simulink model "Compare_AI_kk"  (R2024b)
settings: Solver=ode1  StartTime=0.0  StopTime=2.5  FixedStep=Ts  RelTol=1e-3
PreLoadFcn:
  | Net_improve_init;L=Lac_MV;Tctrl=Ts;
PostLoadFcn:
  | Net_improve_init;L=Lac_MV;Tctrl=Ts;
InitFcn:
  | Net_improve_init;L=Lac_MV;Tctrl=Ts;
values from neighbouring files (symbols this model uses):
  C1 = 3300e-6    (= 0.0033)    [Net_improve_init.m]
  f_cari = 2e4/4.1    (= 4878.04878049)    [Net_improve_init.m]
  fs = 60    [Net_improve_init.m]
  Lac_MV = 0.005*3    (= 0.015)    [Net_improve_init.m]
  Pref = 0.3e6    (= 300000)    [Net_improve_init.m]
  R1 = 1e-3    (= 0.001)    [Net_improve_init.m]
  Rac_MV = 0.1    [Net_improve_init.m]
  Ts = 20e-6    (= 2e-05)    [Net_improve_init.m]
  Vac_peak_MV = Vref*sqrt(2/3)    [Net_improve_init.m]
  Vdc = 3e3    (= 3000)    [Net_improve_init.m]
undefined symbols (not defined in the file or in its folder): dend, DiscIntNeverNeededParam, numd
libraries: powerlib_extras x15, spsControlledVoltageSourceLib x14, spsCurrentMeasurementLib x8, spsGroundLib x7, spsSeriesRLCBranchLib x7, spsVoltageMeasurementLib x6, spsThreePhaseVIMeasurementLib x5, spsControlledCurrentSourceLib x3, spsIdealSwitchLib x3, spsPower3phInstantaneousLib x3, simulink x3, spsThreePhaseSeriesRLCBranchLib x2
(part 2 of 2)

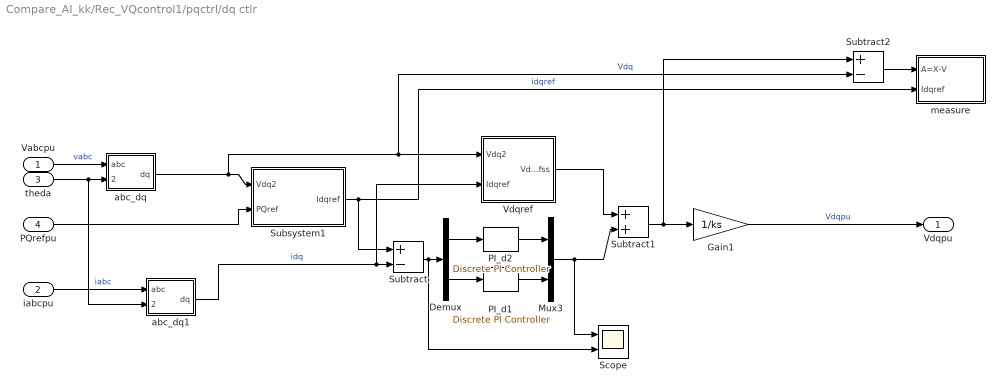
== system Compare_AI_kk/Rec_VQcontrol1/pqctrl/dq ctlr ==
  Vabcpu : Inport
  iabcpu : Inport  Port=2
  theda : Inport  Port=3
  PQrefpu : Inport  Port=4
  Demux : Demux  Outputs=2
  Gain1 : Gain  Gain=1/ks
  Mux3 : Mux  Inputs=2
  PI_d1 : powerlib_extras/Discrete  Control Blocks/Discrete PI Controller  Kp=Kp(1)  Ki=Kp(2)  Par_Limits=[1 -1]*0.15  Init=0  Ts=Ts
  PI_d2 : powerlib_extras/Discrete  Control Blocks/Discrete PI Controller  Kp=Kd(1)  Ki=Kd(2)  Par_Limits=[1 -1]*0.25  Init=0  Ts=Ts
  Scope : Scope  NumInputPorts=2
  Subsystem1 : Subsystem
  Subtract : Sum  Inputs=+-
  Subtract1 : Sum
  Subtract2 : Sum  Inputs=+-
  Vdqref : Subsystem
  abc_dq : Subsystem
  abc_dq1 : Subsystem
  measure : Subsystem
  Vdqpu : Outport  VectorParamsAs1DForOutWhenUnconnected=off
  wires:
  Subtract2/1 -> measure/1(A=X-V)
  Subsystem1/1(Idqref) -> measure/2(Idqref), Subtract/1  "idqref"
  abc_dq/1(dq) -> Subtract2/2, Vdqref/1(Vdq2), Subsystem1/1(Vdq2)  "Vdq"
  abc_dq1/1(dq) -> Vdqref/2(Idqref), Subtract/2  "idq"
  Subtract/1 -> Scope/2, Demux/1
  Demux/1 -> PI_d2/1
  Demux/2 -> PI_d1/1
  Vdqref/1(Vdqrefss) -> Subtract1/1
  PI_d2/1 -> Mux3/1
  PI_d1/1 -> Mux3/2
  Mux3/1 -> Scope/1, Subtract1/2
  Subtract1/1 -> Subtract2/1, Gain1/1
  Vabcpu/1 -> abc_dq/1(abc)  "vabc"
  theda/1 -> abc_dq/2(theta), abc_dq1/2(theta)
  PQrefpu/1 -> Subsystem1/2(PQref)
  iabcpu/1 -> abc_dq1/1(abc)  "iabc"
  Gain1/1 -> Vdqpu/1  "Vdqpu"

== system Compare_AI_kk/Rec_VQcontrol1/pqctrl/dq->abc ==
  note: Va= Vd*sinwt + Vq*cos(wt) + Vo
  note: Vb= Vd*sin(wt-2pi/3) + Vq*cos(wt-2pi/3) + Vo
  note: Vc= Vd*sin(wt+2pi/3) + Vq*cos(wt+2pi/3) + Vo
  dq : Inport
  theda : Inport  Port=2
  Fcn : Fcn  Expr=(u(1)*sin(u(3))+u(2)*cos(u(3)))
  Fcn1 : Fcn  Expr=(u(1)*sin(u(3)-2*pi/3)+u(2)*cos(u(3)-2*pi/3))
  Fcn2 : Fcn  Expr=(u(1)*sin(u(3)+2*pi/3)+u(2)*cos(u(3)+2*pi/3))
  Mux1 : Mux  Inputs=2
  Mux3 : Mux  Inputs=3
  abc : Outport  VectorParamsAs1DForOutWhenUnconnected=off
  wires:
  Fcn2/1 -> Mux3/3
  Fcn1/1 -> Mux3/2
  Fcn/1 -> Mux3/1
  Mux1/1 -> Fcn/1, Fcn2/1, Fcn1/1
  dq/1 -> Mux1/1
  theda/1 -> Mux1/2
  Mux3/1 -> abc/1  "abc"

== system Compare_AI_kk/Rec_VQcontrol1/pqctrl/satuation on amplitute  ==
  Vdq : Inport
  limitVdq : Inport  Port=2
  "Bias important; cancel delay in control cycle, so the PI(error) is zero, other wise PI(errer) is bais, which could over limit" : Bias  Bias=nadv*Ts*2*pi*frq  SaturateOnIntegerOverflow=off
  Complex to Magnitude-Angle : ComplexToMagnitudeAngle
  Complex to Real-Imag : ComplexToRealImag
  Demux1 : Demux  Outputs=2
  Gain : Gain  Gain=-1
  Magnitude-Angle to Complex : MagnitudeAngleToComplex
  Mux4 : Mux  Inputs=2
  Real-Imag to Complex : RealImagToComplex
  Saturation Dynamic : simulink/Discontinuities/Saturation Dynamic  OutMin=[]  OutMax=[]  OutDataTypeStr=Inherit: Same as second input  OutDataType=fixdt(1, 16)  OutScaling=2^-10  DoSatur=off
  Out1 : Outport  VectorParamsAs1DForOutWhenUnconnected=off
  wires:
  "Bias important; cancel delay in control cycle, so the PI(error) is zero, other wise PI(errer) is bais, which could over limit"/1 -> Magnitude-Angle to Complex/2
  Gain/1 -> Saturation Dynamic/3
  limitVdq/1 -> Saturation Dynamic/1, Gain/1
  Complex to Magnitude-Angle/1 -> Saturation Dynamic/2
  Saturation Dynamic/1 -> Magnitude-Angle to Complex/1
  Demux1/1 -> Real-Imag to Complex/1
  Demux1/2 -> Real-Imag to Complex/2
  Real-Imag to Complex/1 -> Complex to Magnitude-Angle/1
  Complex to Magnitude-Angle/2 -> "Bias important; cancel delay in control cycle, so the PI(error) is zero, other wise PI(errer) is bais, which could over limit"/1
  Magnitude-Angle to Complex/1 -> Complex to Real-Imag/1
  Complex to Real-Imag/2 -> Mux4/2
  Complex to Real-Imag/1 -> Mux4/1
  Mux4/1 -> Out1/1
  Vdq/1 -> Demux1/1

== system Compare_AI_kk/Rec_VQcontrol2/Vdc ctrl/Vdc_ctrler1 ==
  Vcap : Inport
  Add2 : Sum  Inputs=+-
  PI_d2 : Subsystem  AncestorBlock=|  DialogController=POWERSYS.PowerSysDialog  mask(Discrete PI Controller){Kp=Kvdc(1), Ki=Kvdc(2), Par_Limits=[1 -1]*1, Init=0, Ts=Ts}
      | powerlib_extras/Discrete 
      | Control Blocks/Discrete
      | PI Controller
      mask prompts: Kp "Proportional gain (Kp):"; Ki "Integral gain (Ki):"; Par_Limits "Output limits: [ Upper   Lower ]"; Init "Output initial value:"; Ts "Sample time:"
      mask help: This block implements a discrete PI controller.
      mask init:
      | UpperLimit=Par_Limits(1);
      | LowerLimit=Par_Limits(2);
      | power_initmask();
      mask Help: This block is part of a subset of blocks in the Extras library that does not have documentation associated with it, other than the block mask description.
      mask Display: disp('PI');
  Saturation : Saturate  UpperLimit=0.1  LowerLimit=-0.1
      settings: AttributesFormatString=%<LowerLimit>~%<UpperLimit>
  Vdcpuref : Constant
  Vdctrl : Scope  NumInputPorts=2
  delP : Outport  OutputWhenDisabled=reset  InitialOutput=[0]  VectorParamsAs1DForOutWhenUnconnected=off
  wires:
  PI_d2/1(Out) -> delP/1, Vdctrl/2  "PIVdc"
  Saturation/1 -> PI_d2/1(Error)
  Vdcpuref/1 -> Add2/2
  Vcap/1 -> Add2/1, Vdctrl/1
  Add2/1 -> Saturation/1  "delVdc"

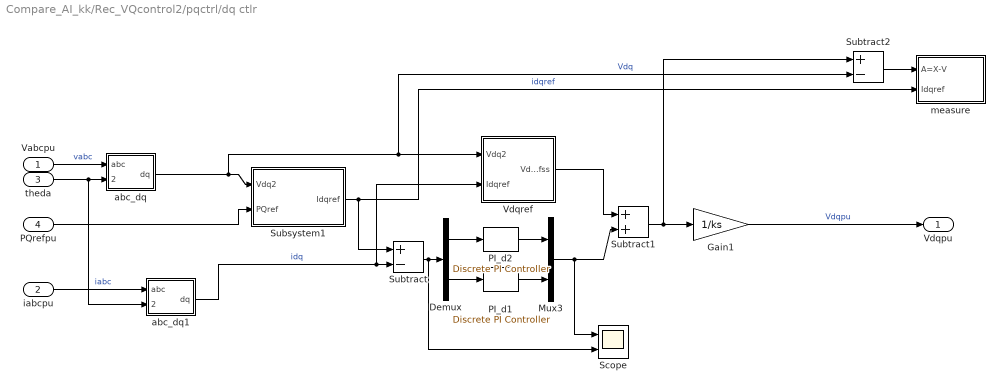
== system Compare_AI_kk/Rec_VQcontrol2/pqctrl/dq ctlr ==
  Vabcpu : Inport
  iabcpu : Inport  Port=2
  theda : Inport  Port=3
  PQrefpu : Inport  Port=4
  Demux : Demux  Outputs=2
  Gain1 : Gain  Gain=1/ks
  Mux3 : Mux  Inputs=2
  PI_d1 : powerlib_extras/Discrete  Control Blocks/Discrete PI Controller  Kp=Kp(1)  Ki=Kp(2)  Par_Limits=[1 -1]*0.15  Init=0  Ts=Ts
  PI_d2 : powerlib_extras/Discrete  Control Blocks/Discrete PI Controller  Kp=Kd(1)  Ki=Kd(2)  Par_Limits=[1 -1]*0.25  Init=0  Ts=Ts
  Scope : Scope  NumInputPorts=2
  Subsystem1 : Subsystem
  Subtract : Sum  Inputs=+-
  Subtract1 : Sum
  Subtract2 : Sum  Inputs=+-
  Vdqref : Subsystem
  abc_dq : Subsystem
  abc_dq1 : Subsystem
  measure : Subsystem
  Vdqpu : Outport  VectorParamsAs1DForOutWhenUnconnected=off
  wires:
  Subtract2/1 -> measure/1(A=X-V)
  Subsystem1/1(Idqref) -> measure/2(Idqref), Subtract/1  "idqref"
  abc_dq/1(dq) -> Subtract2/2, Vdqref/1(Vdq2), Subsystem1/1(Vdq2)  "Vdq"
  abc_dq1/1(dq) -> Vdqref/2(Idqref), Subtract/2  "idq"
  Subtract/1 -> Scope/2, Demux/1
  Demux/1 -> PI_d2/1
  Demux/2 -> PI_d1/1
  Vdqref/1(Vdqrefss) -> Subtract1/1
  PI_d2/1 -> Mux3/1
  PI_d1/1 -> Mux3/2
  Mux3/1 -> Scope/1, Subtract1/2
  Subtract1/1 -> Subtract2/1, Gain1/1
  Vabcpu/1 -> abc_dq/1(abc)  "vabc"
  theda/1 -> abc_dq/2(theta), abc_dq1/2(theta)
  PQrefpu/1 -> Subsystem1/2(PQref)
  iabcpu/1 -> abc_dq1/1(abc)  "iabc"
  Gain1/1 -> Vdqpu/1  "Vdqpu"

== system Compare_AI_kk/Rec_VQcontrol2/pqctrl/dq->abc ==
  note: Va= Vd*sinwt + Vq*cos(wt) + Vo
  note: Vb= Vd*sin(wt-2pi/3) + Vq*cos(wt-2pi/3) + Vo
  note: Vc= Vd*sin(wt+2pi/3) + Vq*cos(wt+2pi/3) + Vo
  dq : Inport
  theda : Inport  Port=2
  Fcn : Fcn  Expr=(u(1)*sin(u(3))+u(2)*cos(u(3)))
  Fcn1 : Fcn  Expr=(u(1)*sin(u(3)-2*pi/3)+u(2)*cos(u(3)-2*pi/3))
  Fcn2 : Fcn  Expr=(u(1)*sin(u(3)+2*pi/3)+u(2)*cos(u(3)+2*pi/3))
  Mux1 : Mux  Inputs=2
  Mux3 : Mux  Inputs=3
  abc : Outport  VectorParamsAs1DForOutWhenUnconnected=off
  wires:
  Fcn2/1 -> Mux3/3
  Fcn1/1 -> Mux3/2
  Fcn/1 -> Mux3/1
  Mux1/1 -> Fcn/1, Fcn2/1, Fcn1/1
  dq/1 -> Mux1/1
  theda/1 -> Mux1/2
  Mux3/1 -> abc/1  "abc"

== system Compare_AI_kk/Rec_VQcontrol2/pqctrl/satuation on amplitute  ==
  Vdq : Inport
  limitVdq : Inport  Port=2
  "Bias important; cancel delay in control cycle, so the PI(error) is zero, other wise PI(errer) is bais, which could over limit" : Bias  Bias=nadv*Ts*2*pi*frq  SaturateOnIntegerOverflow=off
  Complex to Magnitude-Angle : ComplexToMagnitudeAngle
  Complex to Real-Imag : ComplexToRealImag
  Demux1 : Demux  Outputs=2
  Gain : Gain  Gain=-1
  Magnitude-Angle to Complex : MagnitudeAngleToComplex
  Mux4 : Mux  Inputs=2
  Real-Imag to Complex : RealImagToComplex
  Saturation Dynamic : simulink/Discontinuities/Saturation Dynamic  OutMin=[]  OutMax=[]  OutDataTypeStr=Inherit: Same as second input  OutDataType=fixdt(1, 16)  OutScaling=2^-10  DoSatur=off
  Out1 : Outport  VectorParamsAs1DForOutWhenUnconnected=off
  wires:
  "Bias important; cancel delay in control cycle, so the PI(error) is zero, other wise PI(errer) is bais, which could over limit"/1 -> Magnitude-Angle to Complex/2
  Gain/1 -> Saturation Dynamic/3
  limitVdq/1 -> Saturation Dynamic/1, Gain/1
  Complex to Magnitude-Angle/1 -> Saturation Dynamic/2
  Saturation Dynamic/1 -> Magnitude-Angle to Complex/1
  Demux1/1 -> Real-Imag to Complex/1
  Demux1/2 -> Real-Imag to Complex/2
  Real-Imag to Complex/1 -> Complex to Magnitude-Angle/1
  Complex to Magnitude-Angle/2 -> "Bias important; cancel delay in control cycle, so the PI(error) is zero, other wise PI(errer) is bais, which could over limit"/1
  Magnitude-Angle to Complex/1 -> Complex to Real-Imag/1
  Complex to Real-Imag/2 -> Mux4/2
  Complex to Real-Imag/1 -> Mux4/1
  Mux4/1 -> Out1/1
  Vdq/1 -> Demux1/1

== system Compare_AI_kk/Rec_VQcontrol3/Vdc ctrl/Vdc_ctrler1 ==
  Vcap : Inport
  Add2 : Sum  Inputs=+-
  PI_d2 : Subsystem  AncestorBlock=|  DialogController=POWERSYS.PowerSysDialog  mask(Discrete PI Controller){Kp=Kvdc(1), Ki=Kvdc(2), Par_Limits=[1 -1]*1, Init=0, Ts=Ts}
      | powerlib_extras/Discrete 
      | Control Blocks/Discrete
      | PI Controller
      mask prompts: Kp "Proportional gain (Kp):"; Ki "Integral gain (Ki):"; Par_Limits "Output limits: [ Upper   Lower ]"; Init "Output initial value:"; Ts "Sample time:"
      mask help: This block implements a discrete PI controller.
      mask init:
      | UpperLimit=Par_Limits(1);
      | LowerLimit=Par_Limits(2);
      | power_initmask();
      mask Help: This block is part of a subset of blocks in the Extras library that does not have documentation associated with it, other than the block mask description.
      mask Display: disp('PI');
  Saturation : Saturate  UpperLimit=0.1  LowerLimit=-0.1
      settings: AttributesFormatString=%<LowerLimit>~%<UpperLimit>
  Vdcpuref : Constant
  Vdctrl : Scope  NumInputPorts=2
  delP : Outport  OutputWhenDisabled=reset  InitialOutput=[0]  VectorParamsAs1DForOutWhenUnconnected=off
  wires:
  PI_d2/1(Out) -> delP/1, Vdctrl/2  "PIVdc"
  Saturation/1 -> PI_d2/1(Error)
  Vdcpuref/1 -> Add2/2
  Vcap/1 -> Add2/1, Vdctrl/1
  Add2/1 -> Saturation/1  "delVdc"

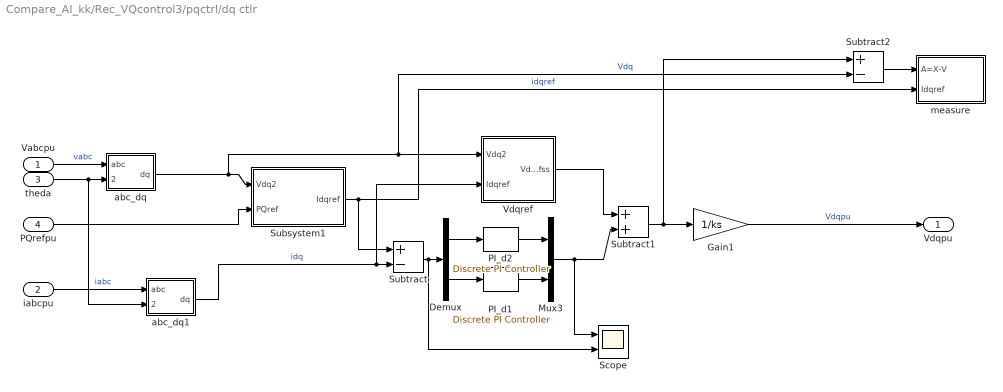
== system Compare_AI_kk/Rec_VQcontrol3/pqctrl/dq ctlr ==
  Vabcpu : Inport
  iabcpu : Inport  Port=2
  theda : Inport  Port=3
  PQrefpu : Inport  Port=4
  Demux : Demux  Outputs=2
  Gain1 : Gain  Gain=1/ks
  Mux3 : Mux  Inputs=2
  PI_d1 : powerlib_extras/Discrete  Control Blocks/Discrete PI Controller  Kp=Kp(1)  Ki=Kp(2)  Par_Limits=[1 -1]*0.15  Init=0  Ts=Ts
  PI_d2 : powerlib_extras/Discrete  Control Blocks/Discrete PI Controller  Kp=Kd(1)  Ki=Kd(2)  Par_Limits=[1 -1]*0.25  Init=0  Ts=Ts
  Scope : Scope  NumInputPorts=2
  Subsystem1 : Subsystem
  Subtract : Sum  Inputs=+-
  Subtract1 : Sum
  Subtract2 : Sum  Inputs=+-
  Vdqref : Subsystem
  abc_dq : Subsystem
  abc_dq1 : Subsystem
  measure : Subsystem
  Vdqpu : Outport  VectorParamsAs1DForOutWhenUnconnected=off
  wires:
  Subtract2/1 -> measure/1(A=X-V)
  Subsystem1/1(Idqref) -> measure/2(Idqref), Subtract/1  "idqref"
  abc_dq/1(dq) -> Subtract2/2, Vdqref/1(Vdq2), Subsystem1/1(Vdq2)  "Vdq"
  abc_dq1/1(dq) -> Vdqref/2(Idqref), Subtract/2  "idq"
  Subtract/1 -> Scope/2, Demux/1
  Demux/1 -> PI_d2/1
  Demux/2 -> PI_d1/1
  Vdqref/1(Vdqrefss) -> Subtract1/1
  PI_d2/1 -> Mux3/1
  PI_d1/1 -> Mux3/2
  Mux3/1 -> Scope/1, Subtract1/2
  Subtract1/1 -> Subtract2/1, Gain1/1
  Vabcpu/1 -> abc_dq/1(abc)  "vabc"
  theda/1 -> abc_dq/2(theta), abc_dq1/2(theta)
  PQrefpu/1 -> Subsystem1/2(PQref)
  iabcpu/1 -> abc_dq1/1(abc)  "iabc"
  Gain1/1 -> Vdqpu/1  "Vdqpu"

== system Compare_AI_kk/Rec_VQcontrol3/pqctrl/dq->abc ==
  note: Va= Vd*sinwt + Vq*cos(wt) + Vo
  note: Vb= Vd*sin(wt-2pi/3) + Vq*cos(wt-2pi/3) + Vo
  note: Vc= Vd*sin(wt+2pi/3) + Vq*cos(wt+2pi/3) + Vo
  dq : Inport
  theda : Inport  Port=2
  Fcn : Fcn  Expr=(u(1)*sin(u(3))+u(2)*cos(u(3)))
  Fcn1 : Fcn  Expr=(u(1)*sin(u(3)-2*pi/3)+u(2)*cos(u(3)-2*pi/3))
  Fcn2 : Fcn  Expr=(u(1)*sin(u(3)+2*pi/3)+u(2)*cos(u(3)+2*pi/3))
  Mux1 : Mux  Inputs=2
  Mux3 : Mux  Inputs=3
  abc : Outport  VectorParamsAs1DForOutWhenUnconnected=off
  wires:
  Fcn2/1 -> Mux3/3
  Fcn1/1 -> Mux3/2
  Fcn/1 -> Mux3/1
  Mux1/1 -> Fcn/1, Fcn2/1, Fcn1/1
  dq/1 -> Mux1/1
  theda/1 -> Mux1/2
  Mux3/1 -> abc/1  "abc"

== system Compare_AI_kk/Rec_VQcontrol3/pqctrl/satuation on amplitute  ==
  Vdq : Inport
  limitVdq : Inport  Port=2
  "Bias important; cancel delay in control cycle, so the PI(error) is zero, other wise PI(errer) is bais, which could over limit" : Bias  Bias=nadv*Ts*2*pi*frq  SaturateOnIntegerOverflow=off
  Complex to Magnitude-Angle : ComplexToMagnitudeAngle
  Complex to Real-Imag : ComplexToRealImag
  Demux1 : Demux  Outputs=2
  Gain : Gain  Gain=-1
  Magnitude-Angle to Complex : MagnitudeAngleToComplex
  Mux4 : Mux  Inputs=2
  Real-Imag to Complex : RealImagToComplex
  Saturation Dynamic : simulink/Discontinuities/Saturation Dynamic  OutMin=[]  OutMax=[]  OutDataTypeStr=Inherit: Same as second input  OutDataType=fixdt(1, 16)  OutScaling=2^-10  DoSatur=off
  Out1 : Outport  VectorParamsAs1DForOutWhenUnconnected=off
  wires:
  "Bias important; cancel delay in control cycle, so the PI(error) is zero, other wise PI(errer) is bais, which could over limit"/1 -> Magnitude-Angle to Complex/2
  Gain/1 -> Saturation Dynamic/3
  limitVdq/1 -> Saturation Dynamic/1, Gain/1
  Complex to Magnitude-Angle/1 -> Saturation Dynamic/2
  Saturation Dynamic/1 -> Magnitude-Angle to Complex/1
  Demux1/1 -> Real-Imag to Complex/1
  Demux1/2 -> Real-Imag to Complex/2
  Real-Imag to Complex/1 -> Complex to Magnitude-Angle/1
  Complex to Magnitude-Angle/2 -> "Bias important; cancel delay in control cycle, so the PI(error) is zero, other wise PI(errer) is bais, which could over limit"/1
  Magnitude-Angle to Complex/1 -> Complex to Real-Imag/1
  Complex to Real-Imag/2 -> Mux4/2
  Complex to Real-Imag/1 -> Mux4/1
  Mux4/1 -> Out1/1
  Vdq/1 -> Demux1/1

== system Compare_AI_kk/Rec_VQcontrol1/Vdc ctrl/Vdc_ctrler1/PI_d2 ==
  note: Discrete PID Controller
  note: Pierre Giroux, Gilbert Sybille
      | Power System Simulation Laboratory
      | IREQ, Hydro-Quebc
  Error : Inport  SampleTime=Ts
  Discrete-Time Integrator : DiscreteIntegrator  InitialCondition=Init  SampleTime=Ts  LimitOutput=on  UpperSaturationLimit=UpperLimit  LowerSaturationLimit=LowerLimit  ICPrevOutput=DiscIntNeverNeededParam  ICPrevScaledInput=DiscIntNeverNeededParam
  Kp4 : Gain  Gain=Kp  SaturateOnIntegerOverflow=on  SampleTime=Ts  OutDataTypeStr=Inherit: Same as input  ParamDataTypeStr=Inherit: Same as input
  Kp5 : Gain  Gain=Ki  SaturateOnIntegerOverflow=on  SampleTime=Ts  OutDataTypeStr=Inherit: Same as input  ParamDataTypeStr=Inherit: Same as input
  Saturation2 : Saturate  UpperLimit=UpperLimit  LowerLimit=LowerLimit  SampleTime=Ts
  Sum6 : Sum  InputSameDT=on  SaturateOnIntegerOverflow=on  SampleTime=Ts  OutDataTypeStr=Inherit: Same as first input
  Zero-Order Hold : ZeroOrderHold  SampleTime=Ts
  Out : Outport  SampleTime=Ts  InitialOutput=0  VectorParamsAs1DForOutWhenUnconnected=off
  wires:
  Zero-Order Hold/1 -> Sum6/1  "prop"
  Saturation2/1 -> Out/1
  Discrete-Time Integrator/1 -> Sum6/2  "int"
  Kp4/1 -> Zero-Order Hold/1
  Kp5/1 -> Discrete-Time Integrator/1
  Sum6/1 -> Saturation2/1
  Error/1 -> Kp5/1, Kp4/1

== system Compare_AI_kk/Rec_VQcontrol1/pqctrl/dq ctlr/Subsystem1 ==
  Vdq2 : Inport
  PQref : Inport  Port=2
  Fcn7 : Fcn  Expr=(u[1] *u[4]+u[2]*u[5])/u[3]
  Fcn8 : Fcn  Expr=(u[2] *u[4]-u[1]*u[5])/u[3]
  Fcn9 : Fcn  Expr=(u[1] ^2+u[2]^2)
  Mux3 : Mux  Inputs=[2 1 2]
  Mux4 : Mux  Inputs=2
  Saturation : Saturate  UpperLimit=inf  LowerLimit=0.01
  Saturation1 : Saturate  UpperLimit=1.5  LowerLimit=-1.5
  Idqref : Outport  VectorParamsAs1DForOutWhenUnconnected=off
  wires:
  Saturation1/1 -> Idqref/1
  Vdq2/1 -> Fcn9/1, Mux3/1
  Mux3/1 -> Fcn8/1, Fcn7/1
  Fcn9/1 -> Saturation/1
  Fcn7/1 -> Mux4/1
  Fcn8/1 -> Mux4/2
  Mux4/1 -> Saturation1/1  "Idqref"
  PQref/1 -> Mux3/3
  Saturation/1 -> Mux3/2

== system Compare_AI_kk/Rec_VQcontrol1/pqctrl/dq ctlr/Vdqref ==
  Vdq2 : Inport
  Idqref : Inport  Port=2
  Display : Display
      settings: Decimation=50
  Fcn7 : Fcn  Expr=(u[2] +u[4]*u[5]+u[3]*u[6])
  Fcn8 : Fcn  Expr=(u[1] +u[3]*u[5]-u[4]*u[6])
  Lxpu : Constant  Value=Lxpu
  Mux3 : Mux
  Mux4 : Mux  Inputs=2
  Rxpu : Constant  Value=Rxpu
  Vdqrefss : Outport  VectorParamsAs1DForOutWhenUnconnected=off
  wires:
  Lxpu/1 -> Mux3/4
  Rxpu/1 -> Mux3/3
  Mux3/1 -> Display/1, Fcn8/1, Fcn7/1
  Fcn8/1 -> Mux4/1  "Vdref"
  Fcn7/1 -> Mux4/2  "Vqref"
  Vdq2/1 -> Mux3/1
  Idqref/1 -> Mux3/2
  Mux4/1 -> Vdqrefss/1

== system Compare_AI_kk/Rec_VQcontrol1/pqctrl/dq ctlr/abc_dq ==
  abc : Inport
  theta : Inport  Port=2
  Mux2 : Mux  Inputs=2
  Selector3 : Selector  InputPortWidth=3  IndexOptions=Index vector (dialog)  Indices=[1 2]  OutputSizes=1
  Trigonometric Function2 : Trigonometry
  Trigonometric Function3 : Trigonometry  Operator=cos
  abc/dq1 : powerlib_extras/Measurements/abc_to_dq0 Transformation
  dq : Outport  VectorParamsAs1DForOutWhenUnconnected=off
  wires:
  abc/1 -> abc/dq1/1
  Selector3/1 -> dq/1
  abc/dq1/1 -> Selector3/1
  Mux2/1 -> abc/dq1/2
  theta/1 -> Trigonometric Function3/1, Trigonometric Function2/1
  Trigonometric Function2/1 -> Mux2/1
  Trigonometric Function3/1 -> Mux2/2

== system Compare_AI_kk/Rec_VQcontrol1/pqctrl/dq ctlr/abc_dq1 ==
  abc : Inport
  theta : Inport  Port=2
  Mux2 : Mux  Inputs=2
  Selector3 : Selector  InputPortWidth=3  IndexOptions=Index vector (dialog)  Indices=[1 2]  OutputSizes=1
  Trigonometric Function2 : Trigonometry
  Trigonometric Function3 : Trigonometry  Operator=cos
  abc/dq1 : powerlib_extras/Measurements/abc_to_dq0 Transformation
  dq : Outport  VectorParamsAs1DForOutWhenUnconnected=off
  wires:
  Trigonometric Function3/1 -> Mux2/2
  Trigonometric Function2/1 -> Mux2/1
  theta/1 -> Trigonometric Function2/1, Trigonometric Function3/1
  Mux2/1 -> abc/dq1/2
  abc/dq1/1 -> Selector3/1
  Selector3/1 -> dq/1
  abc/1 -> abc/dq1/1

== system Compare_AI_kk/Rec_VQcontrol1/pqctrl/dq ctlr/measure ==
  note: this is to validate Rxpu and Lxpu which make PI(error) almost zero,
      | i.e. the delay is properly set
      |
      | or to calculate Rxpu and Lxpu which make PI(error) zero
      | when input are in steady state
      |
      | when change the P,Q ref,
      | the results should be same if delay is properly cancelled
  A=X-V : Inport
  Idqref : Inport  Port=2
  Display1 : Display
      settings: Decimation=200
  Fcn7 : Fcn  Expr=(u[2] *u[3]-u[1]*u[4])/(u[3]^2+u[4]^2)
  Fcn8 : Fcn  Expr=(u[1] *u[3]+u[2]*u[4])/(u[3]^2+u[4]^2)
  Mux3 : Mux  Inputs=2
  Mux4 : Mux  Inputs=2
  wires:
  Mux3/1 -> Fcn8/1, Fcn7/1
  Fcn8/1 -> Mux4/1  "Rxpu"
  Fcn7/1 -> Mux4/2  "Lxpu"
  A=X-V/1 -> Mux3/1
  Idqref/1 -> Mux3/2
  Mux4/1 -> Display1/1

== system Compare_AI_kk/Rec_VQcontrol2/Vdc ctrl/Vdc_ctrler1/PI_d2 ==
  note: Discrete PID Controller
  note: Pierre Giroux, Gilbert Sybille
      | Power System Simulation Laboratory
      | IREQ, Hydro-Quebc
  Error : Inport  SampleTime=Ts
  Discrete-Time Integrator : DiscreteIntegrator  InitialCondition=Init  SampleTime=Ts  LimitOutput=on  UpperSaturationLimit=UpperLimit  LowerSaturationLimit=LowerLimit  ICPrevOutput=DiscIntNeverNeededParam  ICPrevScaledInput=DiscIntNeverNeededParam
  Kp4 : Gain  Gain=Kp  SaturateOnIntegerOverflow=on  SampleTime=Ts  OutDataTypeStr=Inherit: Same as input  ParamDataTypeStr=Inherit: Same as input
  Kp5 : Gain  Gain=Ki  SaturateOnIntegerOverflow=on  SampleTime=Ts  OutDataTypeStr=Inherit: Same as input  ParamDataTypeStr=Inherit: Same as input
  Saturation2 : Saturate  UpperLimit=UpperLimit  LowerLimit=LowerLimit  SampleTime=Ts
  Sum6 : Sum  InputSameDT=on  SaturateOnIntegerOverflow=on  SampleTime=Ts  OutDataTypeStr=Inherit: Same as first input
  Zero-Order Hold : ZeroOrderHold  SampleTime=Ts
  Out : Outport  SampleTime=Ts  InitialOutput=0  VectorParamsAs1DForOutWhenUnconnected=off
  wires:
  Zero-Order Hold/1 -> Sum6/1  "prop"
  Saturation2/1 -> Out/1
  Discrete-Time Integrator/1 -> Sum6/2  "int"
  Kp4/1 -> Zero-Order Hold/1
  Kp5/1 -> Discrete-Time Integrator/1
  Sum6/1 -> Saturation2/1
  Error/1 -> Kp5/1, Kp4/1

== system Compare_AI_kk/Rec_VQcontrol2/pqctrl/dq ctlr/Subsystem1 ==
  Vdq2 : Inport
  PQref : Inport  Port=2
  Fcn7 : Fcn  Expr=(u[1] *u[4]+u[2]*u[5])/u[3]
  Fcn8 : Fcn  Expr=(u[2] *u[4]-u[1]*u[5])/u[3]
  Fcn9 : Fcn  Expr=(u[1] ^2+u[2]^2)
  Mux3 : Mux  Inputs=[2 1 2]
  Mux4 : Mux  Inputs=2
  Saturation : Saturate  UpperLimit=inf  LowerLimit=0.01
  Saturation1 : Saturate  UpperLimit=1.5  LowerLimit=-1.5
  Idqref : Outport  VectorParamsAs1DForOutWhenUnconnected=off
  wires:
  Saturation1/1 -> Idqref/1
  Vdq2/1 -> Fcn9/1, Mux3/1
  Mux3/1 -> Fcn8/1, Fcn7/1
  Fcn9/1 -> Saturation/1
  Fcn7/1 -> Mux4/1
  Fcn8/1 -> Mux4/2
  Mux4/1 -> Saturation1/1  "Idqref"
  PQref/1 -> Mux3/3
  Saturation/1 -> Mux3/2

== system Compare_AI_kk/Rec_VQcontrol2/pqctrl/dq ctlr/Vdqref ==
  Vdq2 : Inport
  Idqref : Inport  Port=2
  Display : Display
      settings: Decimation=50
  Fcn7 : Fcn  Expr=(u[2] +u[4]*u[5]+u[3]*u[6])
  Fcn8 : Fcn  Expr=(u[1] +u[3]*u[5]-u[4]*u[6])
  Lxpu : Constant  Value=Lxpu
  Mux3 : Mux
  Mux4 : Mux  Inputs=2
  Rxpu : Constant  Value=Rxpu
  Vdqrefss : Outport  VectorParamsAs1DForOutWhenUnconnected=off
  wires:
  Lxpu/1 -> Mux3/4
  Rxpu/1 -> Mux3/3
  Mux3/1 -> Display/1, Fcn8/1, Fcn7/1
  Fcn8/1 -> Mux4/1  "Vdref"
  Fcn7/1 -> Mux4/2  "Vqref"
  Vdq2/1 -> Mux3/1
  Idqref/1 -> Mux3/2
  Mux4/1 -> Vdqrefss/1

== system Compare_AI_kk/Rec_VQcontrol2/pqctrl/dq ctlr/abc_dq ==
  abc : Inport
  theta : Inport  Port=2
  Mux2 : Mux  Inputs=2
  Selector3 : Selector  InputPortWidth=3  IndexOptions=Index vector (dialog)  Indices=[1 2]  OutputSizes=1
  Trigonometric Function2 : Trigonometry
  Trigonometric Function3 : Trigonometry  Operator=cos
  abc/dq1 : powerlib_extras/Measurements/abc_to_dq0 Transformation
  dq : Outport  VectorParamsAs1DForOutWhenUnconnected=off
  wires:
  abc/1 -> abc/dq1/1
  Selector3/1 -> dq/1
  abc/dq1/1 -> Selector3/1
  Mux2/1 -> abc/dq1/2
  theta/1 -> Trigonometric Function3/1, Trigonometric Function2/1
  Trigonometric Function2/1 -> Mux2/1
  Trigonometric Function3/1 -> Mux2/2

== system Compare_AI_kk/Rec_VQcontrol2/pqctrl/dq ctlr/abc_dq1 ==
  abc : Inport
  theta : Inport  Port=2
  Mux2 : Mux  Inputs=2
  Selector3 : Selector  InputPortWidth=3  IndexOptions=Index vector (dialog)  Indices=[1 2]  OutputSizes=1
  Trigonometric Function2 : Trigonometry
  Trigonometric Function3 : Trigonometry  Operator=cos
  abc/dq1 : powerlib_extras/Measurements/abc_to_dq0 Transformation
  dq : Outport  VectorParamsAs1DForOutWhenUnconnected=off
  wires:
  Trigonometric Function3/1 -> Mux2/2
  Trigonometric Function2/1 -> Mux2/1
  theta/1 -> Trigonometric Function2/1, Trigonometric Function3/1
  Mux2/1 -> abc/dq1/2
  abc/dq1/1 -> Selector3/1
  Selector3/1 -> dq/1
  abc/1 -> abc/dq1/1

== system Compare_AI_kk/Rec_VQcontrol2/pqctrl/dq ctlr/measure ==
  note: this is to validate Rxpu and Lxpu which make PI(error) almost zero,
      | i.e. the delay is properly set
      |
      | or to calculate Rxpu and Lxpu which make PI(error) zero
      | when input are in steady state
      |
      | when change the P,Q ref,
      | the results should be same if delay is properly cancelled
  A=X-V : Inport
  Idqref : Inport  Port=2
  Display1 : Display
      settings: Decimation=200
  Fcn7 : Fcn  Expr=(u[2] *u[3]-u[1]*u[4])/(u[3]^2+u[4]^2)
  Fcn8 : Fcn  Expr=(u[1] *u[3]+u[2]*u[4])/(u[3]^2+u[4]^2)
  Mux3 : Mux  Inputs=2
  Mux4 : Mux  Inputs=2
  wires:
  Mux3/1 -> Fcn8/1, Fcn7/1
  Fcn8/1 -> Mux4/1  "Rxpu"
  Fcn7/1 -> Mux4/2  "Lxpu"
  A=X-V/1 -> Mux3/1
  Idqref/1 -> Mux3/2
  Mux4/1 -> Display1/1

== system Compare_AI_kk/Rec_VQcontrol3/Vdc ctrl/Vdc_ctrler1/PI_d2 ==
  note: Discrete PID Controller
  note: Pierre Giroux, Gilbert Sybille
      | Power System Simulation Laboratory
      | IREQ, Hydro-Quebc
  Error : Inport  SampleTime=Ts
  Discrete-Time Integrator : DiscreteIntegrator  InitialCondition=Init  SampleTime=Ts  LimitOutput=on  UpperSaturationLimit=UpperLimit  LowerSaturationLimit=LowerLimit  ICPrevOutput=DiscIntNeverNeededParam  ICPrevScaledInput=DiscIntNeverNeededParam
  Kp4 : Gain  Gain=Kp  SaturateOnIntegerOverflow=on  SampleTime=Ts  OutDataTypeStr=Inherit: Same as input  ParamDataTypeStr=Inherit: Same as input
  Kp5 : Gain  Gain=Ki  SaturateOnIntegerOverflow=on  SampleTime=Ts  OutDataTypeStr=Inherit: Same as input  ParamDataTypeStr=Inherit: Same as input
  Saturation2 : Saturate  UpperLimit=UpperLimit  LowerLimit=LowerLimit  SampleTime=Ts
  Sum6 : Sum  InputSameDT=on  SaturateOnIntegerOverflow=on  SampleTime=Ts  OutDataTypeStr=Inherit: Same as first input
  Zero-Order Hold : ZeroOrderHold  SampleTime=Ts
  Out : Outport  SampleTime=Ts  InitialOutput=0  VectorParamsAs1DForOutWhenUnconnected=off
  wires:
  Zero-Order Hold/1 -> Sum6/1  "prop"
  Saturation2/1 -> Out/1
  Discrete-Time Integrator/1 -> Sum6/2  "int"
  Kp4/1 -> Zero-Order Hold/1
  Kp5/1 -> Discrete-Time Integrator/1
  Sum6/1 -> Saturation2/1
  Error/1 -> Kp5/1, Kp4/1

== system Compare_AI_kk/Rec_VQcontrol3/pqctrl/dq ctlr/Subsystem1 ==
  Vdq2 : Inport
  PQref : Inport  Port=2
  Fcn7 : Fcn  Expr=(u[1] *u[4]+u[2]*u[5])/u[3]
  Fcn8 : Fcn  Expr=(u[2] *u[4]-u[1]*u[5])/u[3]
  Fcn9 : Fcn  Expr=(u[1] ^2+u[2]^2)
  Mux3 : Mux  Inputs=[2 1 2]
  Mux4 : Mux  Inputs=2
  Saturation : Saturate  UpperLimit=inf  LowerLimit=0.01
  Saturation1 : Saturate  UpperLimit=1.5  LowerLimit=-1.5
  Idqref : Outport  VectorParamsAs1DForOutWhenUnconnected=off
  wires:
  Saturation1/1 -> Idqref/1
  Vdq2/1 -> Fcn9/1, Mux3/1
  Mux3/1 -> Fcn8/1, Fcn7/1
  Fcn9/1 -> Saturation/1
  Fcn7/1 -> Mux4/1
  Fcn8/1 -> Mux4/2
  Mux4/1 -> Saturation1/1  "Idqref"
  PQref/1 -> Mux3/3
  Saturation/1 -> Mux3/2

== system Compare_AI_kk/Rec_VQcontrol3/pqctrl/dq ctlr/Vdqref ==
  Vdq2 : Inport
  Idqref : Inport  Port=2
  Display : Display
      settings: Decimation=50
  Fcn7 : Fcn  Expr=(u[2] +u[4]*u[5]+u[3]*u[6])
  Fcn8 : Fcn  Expr=(u[1] +u[3]*u[5]-u[4]*u[6])
  Lxpu : Constant  Value=Lxpu
  Mux3 : Mux
  Mux4 : Mux  Inputs=2
  Rxpu : Constant  Value=Rxpu
  Vdqrefss : Outport  VectorParamsAs1DForOutWhenUnconnected=off
  wires:
  Lxpu/1 -> Mux3/4
  Rxpu/1 -> Mux3/3
  Mux3/1 -> Display/1, Fcn8/1, Fcn7/1
  Fcn8/1 -> Mux4/1  "Vdref"
  Fcn7/1 -> Mux4/2  "Vqref"
  Vdq2/1 -> Mux3/1
  Idqref/1 -> Mux3/2
  Mux4/1 -> Vdqrefss/1

== system Compare_AI_kk/Rec_VQcontrol3/pqctrl/dq ctlr/abc_dq ==
  abc : Inport
  theta : Inport  Port=2
  Mux2 : Mux  Inputs=2
  Selector3 : Selector  InputPortWidth=3  IndexOptions=Index vector (dialog)  Indices=[1 2]  OutputSizes=1
  Trigonometric Function2 : Trigonometry
  Trigonometric Function3 : Trigonometry  Operator=cos
  abc/dq1 : powerlib_extras/Measurements/abc_to_dq0 Transformation
  dq : Outport  VectorParamsAs1DForOutWhenUnconnected=off
  wires:
  abc/1 -> abc/dq1/1
  Selector3/1 -> dq/1
  abc/dq1/1 -> Selector3/1
  Mux2/1 -> abc/dq1/2
  theta/1 -> Trigonometric Function3/1, Trigonometric Function2/1
  Trigonometric Function2/1 -> Mux2/1
  Trigonometric Function3/1 -> Mux2/2

== system Compare_AI_kk/Rec_VQcontrol3/pqctrl/dq ctlr/abc_dq1 ==
  abc : Inport
  theta : Inport  Port=2
  Mux2 : Mux  Inputs=2
  Selector3 : Selector  InputPortWidth=3  IndexOptions=Index vector (dialog)  Indices=[1 2]  OutputSizes=1
  Trigonometric Function2 : Trigonometry
  Trigonometric Function3 : Trigonometry  Operator=cos
  abc/dq1 : powerlib_extras/Measurements/abc_to_dq0 Transformation
  dq : Outport  VectorParamsAs1DForOutWhenUnconnected=off
  wires:
  Trigonometric Function3/1 -> Mux2/2
  Trigonometric Function2/1 -> Mux2/1
  theta/1 -> Trigonometric Function2/1, Trigonometric Function3/1
  Mux2/1 -> abc/dq1/2
  abc/dq1/1 -> Selector3/1
  Selector3/1 -> dq/1
  abc/1 -> abc/dq1/1

== system Compare_AI_kk/Rec_VQcontrol3/pqctrl/dq ctlr/measure ==
  note: this is to validate Rxpu and Lxpu which make PI(error) almost zero,
      | i.e. the delay is properly set
      |
      | or to calculate Rxpu and Lxpu which make PI(error) zero
      | when input are in steady state
      |
      | when change the P,Q ref,
      | the results should be same if delay is properly cancelled
  A=X-V : Inport
  Idqref : Inport  Port=2
  Display1 : Display
      settings: Decimation=200
  Fcn7 : Fcn  Expr=(u[2] *u[3]-u[1]*u[4])/(u[3]^2+u[4]^2)
  Fcn8 : Fcn  Expr=(u[1] *u[3]+u[2]*u[4])/(u[3]^2+u[4]^2)
  Mux3 : Mux  Inputs=2
  Mux4 : Mux  Inputs=2
  wires:
  Mux3/1 -> Fcn8/1, Fcn7/1
  Fcn8/1 -> Mux4/1  "Rxpu"
  Fcn7/1 -> Mux4/2  "Lxpu"
  A=X-V/1 -> Mux3/1
  Idqref/1 -> Mux3/2
  Mux4/1 -> Display1/1

== matlab function Compare_AI_kk/MATLAB Function ==
  data: u input; dz output
function dz = phnode_forward(u)
    % =========================================================
    % 0. 声明持久化变量 (仅在 t=0 时加载和计算一次)
    % =========================================================
    persistent W00 b00 W01 b01 W10 b10 W11 b11 W20 b20 W21 b21 W3 b3 p
    
    if isempty(W00)

        w = coder.load('phnode_weights_3_8.mat');
        
        W00 = double(w.R_module_net_0_0_weight); b00 = double(w.R_module_net_0_0_bias(:));
        W01 = double(w.R_module_net_0_1_weight(:)); b01 = double(w.R_module_net_0_1_bias(:));
        
        W10 = double(w.R_module_net_1_0_weight); b10 = double(w.R_module_net_1_0_bias(:));
        W11 = double(w.R_module_net_1_1_weight(:)); b11 = double(w.R_module_net_1_1_bias(:));
        
        W20 = double(w.R_module_net_2_0_weight); b20 = double(w.R_module_net_2_0_bias(:));
        W21 = double(w.R_module_net_2_1_weight(:)); b21 = double(w.R_module_net_2_1_bias(:));
        
        W3  = double(w.R_module_net_3_weight);   b3  = double(w.R_module_net_3_bias(:));

        p_raw = double(w.Pinv_module_p_raw(:));
        base_scale = [1/3.3e-3; 1/3.3e-3; 1/0.015; 1/0.015; 1/0.015];
        p = log(1.0 + exp(p_raw)) .* base_scale;
    end
    
    % =========================================================
    % 1. 拆解输入向量
    % =========================================================
    z     = double(u(1:5));
    u_ext = double(u(6:10));
    u_sw  = double(u(11:16));
    
    % =========================================================
    % 2. 构造耗散矩阵 R
    % =========================================================
    h = [z; u_sw];
    
    % --- Block 0 ---
    h = W00 * h + b00;
    mu = mean(h); var_h = mean((h - mu).^2);
    h = (h - mu) ./ sqrt(var_h + 1e-5);
    h = W01 .* h + b01;
    h = h ./ (1 + exp(-h)); % SiLU
    
    % --- Block 1 ---    
    h = W10 * h + b10;
    mu = mean(h); var_h = mean((h - mu).^2);
    h = (h - mu) ./ sqrt(var_h + 1e-5);
    h = W11 .* h + b11;
    h = h ./ (1 + exp(-h));
    
    % --- Block 2 ---
    h = W20 * h + b20;
    mu = mean(h); var_h = mean((h - mu).^2);
    h = (h - mu) ./ sqrt(var_h + 1e-5);
    h = W21 .* h + b21;
    h = h ./ (1 + exp(-h));
    
    % --- Output Linear ---
    r_out = W3 * h + b3;   
    r_full = log(1 + exp(r_out)); 
    
    % =========================================================
    % 3. 计算最终输出 dz 稀疏运算
    % =========================================================
    Jz = zeros(5, 1, 'double');
    Jz(1) =  u_sw(1)*z(3) + u_sw(3)*z(4) + u_sw(5)*z(5);
    Jz(2) = -u_sw(2)*z(3) - u_sw(4)*z(4) - u_sw(6)*z(5);
    Jz(3) = -u_sw(1)*z(1) + u_sw(2)*z(2);
    Jz(4) = -u_sw(3)*z(1) + u_sw(4)*z(2);
    Jz(5) = -u_sw(5)*z(1) + u_sw(6)*z(2);
 
    rhs = Jz - r_full .* z + u_ext;
 
    dz = p .* rhs;
end

== matlab function Compare_AI_kk/MATLAB Function1 ==
  data: u input; dz output
function dz = phnode_forward(u)
    % =========================================================
    % 0. 声明持久化变量 (仅在 t=0 时加载和计算一次)
    % =========================================================
    persistent W00 b00 W01 b01 W10 b10 W11 b11 W20 b20 W21 b21 W3 b3 p
    
    if isempty(W00)

        w = coder.load('phnode_weights_3_8.mat');
        
        W00 = double(w.R_module_net_0_0_weight); b00 = double(w.R_module_net_0_0_bias(:));
        W01 = double(w.R_module_net_0_1_weight(:)); b01 = double(w.R_module_net_0_1_bias(:));
        
        W10 = double(w.R_module_net_1_0_weight); b10 = double(w.R_module_net_1_0_bias(:));
        W11 = double(w.R_module_net_1_1_weight(:)); b11 = double(w.R_module_net_1_1_bias(:));
        
        W20 = double(w.R_module_net_2_0_weight); b20 = double(w.R_module_net_2_0_bias(:));
        W21 = double(w.R_module_net_2_1_weight(:)); b21 = double(w.R_module_net_2_1_bias(:));
        
        W3  = double(w.R_module_net_3_weight);   b3  = double(w.R_module_net_3_bias(:));

        p_raw = double(w.Pinv_module_p_raw(:));
        base_scale = [1/3.3e-3; 1/3.3e-3; 1/0.015; 1/0.015; 1/0.015];
        p = log(1.0 + exp(p_raw)) .* base_scale;
    end
    
    % =========================================================
    % 1. 拆解输入向量
    % =========================================================
    z     = double(u(1:5));
    u_ext = double(u(6:10));
    u_sw  = double(u(11:16));
    
    % =========================================================
    % 2. 构造耗散矩阵 R
    % =========================================================
    h = [z; u_sw];
    
    % --- Block 0 ---
    h = W00 * h + b00;
    mu = mean(h); var_h = mean((h - mu).^2);
    h = (h - mu) ./ sqrt(var_h + 1e-5);
    h = W01 .* h + b01;
    h = h ./ (1 + exp(-h)); % SiLU
    
    % --- Block 1 ---    
    h = W10 * h + b10;
    mu = mean(h); var_h = mean((h - mu).^2);
    h = (h - mu) ./ sqrt(var_h + 1e-5);
    h = W11 .* h + b11;
    h = h ./ (1 + exp(-h));
    
    % --- Block 2 ---
    h = W20 * h + b20;
    mu = mean(h); var_h = mean((h - mu).^2);
    h = (h - mu) ./ sqrt(var_h + 1e-5);
    h = W21 .* h + b21;
    h = h ./ (1 + exp(-h));
    
    % --- Output Linear ---
    r_out = W3 * h + b3;   
    r_full = log(1 + exp(r_out)); 
    
    % =========================================================
    % 3. 计算最终输出 dz 稀疏运算
    % =========================================================
    Jz = zeros(5, 1, 'double');
    Jz(1) =  u_sw(1)*z(3) + u_sw(3)*z(4) + u_sw(5)*z(5);
    Jz(2) = -u_sw(2)*z(3) - u_sw(4)*z(4) - u_sw(6)*z(5);
    Jz(3) = -u_sw(1)*z(1) + u_sw(2)*z(2);
    Jz(4) = -u_sw(3)*z(1) + u_sw(4)*z(2);
    Jz(5) = -u_sw(5)*z(1) + u_sw(6)*z(2);
 
    rhs = Jz - r_full .* z + u_ext;
 
    dz = p .* rhs;
end
